simulink model "ex6"  (R2019b)
settings: Solver=VariableStepAuto  StartTime=0.0  StopTime=10.0  RelTol=1e-3
settings Model: Creator=Russty  LastModifiedBy=TimRo
settings DataIOCC: ReturnWorkspaceOutputs=off
settings DebuggingCC: ArithmeticOperatorsInVariantConditions=warning
settings SFSimCC: CustomCodeUndefinedFunction=UseInterfaceOnly

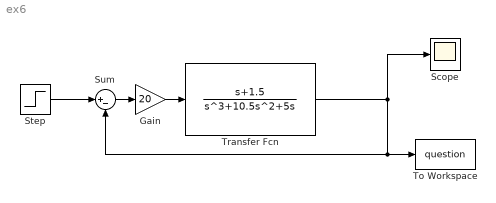
== system ex6 ==
  Gain : Gain  Gain=20
  Scope : Scope
  Step : Step  Time=0  SampleTime=0.001
  Sum : Sum  Inputs=|+-
  To Workspace : ToWorkspace  VariableName=question  SaveFormat=Timeseries  SampleTime=-1
  Transfer Fcn : TransferFcn  Numerator=[1 1.5]  Denominator=[1 10.5 5 0]
  wires:
  Step/1 -> Sum/1
  Transfer Fcn/1 -> Sum/2, To Workspace/1, Scope/1
  Sum/1 -> Gain/1
  Gain/1 -> Transfer Fcn/1
